simulink model "Thrustcontrol"  (R2015a)
settings: Solver=ode3  StartTime=0.0  StopTime=200  FixedStep=0.01  MaxStep=10.0  RelTol=1e-3
values from neighbouring files (symbols this model uses):
  C = [C1;C2;C3;C4;C5;C6]    [initfile.m]    (also in thrustallocationQuadraticFixed.m)
  D = 3.0/100    (= 0.03)    [initfile.m]    (also in thrustallocationQuadraticFixed.m = 0.0411111111111)
  eps_c = 3    [initfile.m]
  epsilon = 0.5    [initfile.m]    (also in thrustallocationPseudo.m = u(10); thrustallocationQuadraticFixed.m = u(10))
  hd = c2d(H1,0.01,'foh')    [initfile.m]
  hd2 = c2d(H2,0.01,'zoh')    [initfile.m]
  I_s = 25000 /747225    (= 0.0334571246947)    [initfile.m]
  k_cc = 1    [initfile.m]
  K_omega = 0.3    [initfile.m]
  Kp = 3.3    [initfile.m]
  Kq = 0.266    [initfile.m]
  Kqr = 0.266    [initfile.m]
  Kt = 0.445    [initfile.m]
  Ktr = 0.445    [initfile.m]
  Max_Acceleration = 5    [initfile.m]
  Max_rotation = 5*sqrt(lambda)    [initfile.m]
  Max_thrust = 0.12    [initfile.m]
  n_c = 5    [initfile.m]
  n_max = (lambda/sqrt(lambda))*170/1.4    [initfile.m]
  p_cc = 0.5    [initfile.m]
  P_max = 2*pi*n_max*Q_max    (= 239.439495498)    [initfile.m]
  pwm_to_shaft_coeff = coeffvalues(PWMToShaft)    [initfile.m]
  pwm_to_thrust_coeff = coeffvalues(PWMToForce)    [initfile.m]
  Q_f0 = 0.3    [initfile.m]
  Q_max = (Kq0*Rho_m*D^5*n_max^2*k)    (= 0.224164584)    [initfile.m]
  r = 0    [initfile.m]    (also in thrustallocationQuadraticFixed.m)
  r_cc = 2    [initfile.m]
  Rho = Rho_m    (= 1000)    [initfile.m]
  shaft_to_pwm_coeff = coeffvalues(ShaftToPWM)    [initfile.m]
  tc = [1;2;0.5]    [initfile.m]    (also in testgd.m = [-1,0,0]'; thrustallocationPseudo.m = [u(1),u(2),u(3)]'; thrustallocationQuadraticFixed.m = [u(1),u(2),u(3)]')
  Thrust_algorithm = 1    [initfile.m]
  thrust_to_pwm_coeff = coeffvalues(ForceToPWM)    [initfile.m]
  Thruster_control = 1    [initfile.m]
  Thruster_lock = 1    [initfile.m]
undefined symbols (not defined in the file or in its folder): Thruster
libraries: simulink x6, simulink_extras x3
(part 1 of 2)
settings Model: CovModelRefEnable=off  Creator=Preben  LastModifiedBy=Preben
settings SolverCC: AlgebraicLoopSolver=LineSearch
settings DataIOCC: SaveFormat=Dataset
settings HardwareCC: ProdBitPerPointer=64  ProdLargestAtomicFloat=Float  ProdIntDivRoundTo=Zero  ProdEndianess=LittleEndian  ProdHWDeviceType=Specified

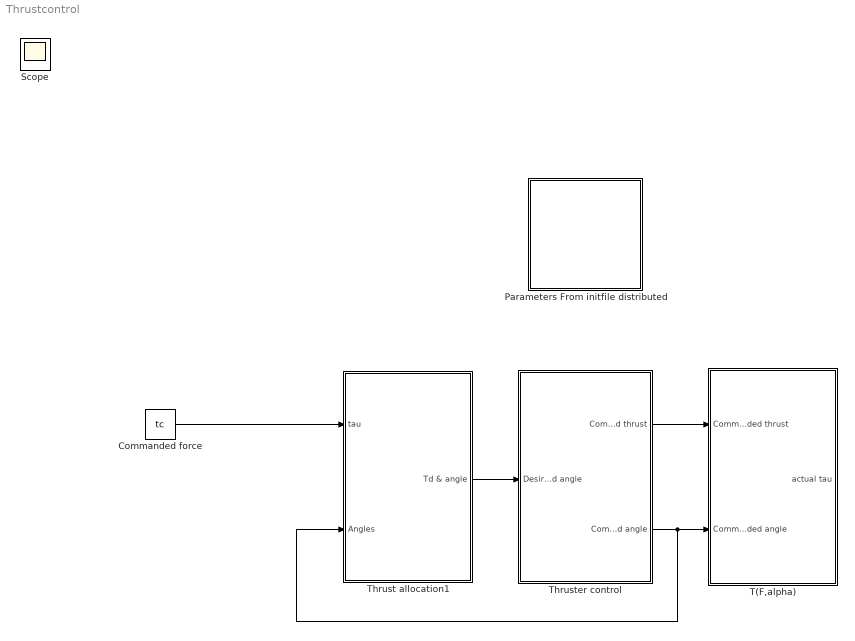
== system Thrustcontrol ==
  Commanded force : Constant  Value=tc
  "Parameters From initfile distributed " : Subsystem
  T(F,alpha) : Subsystem
  Thrust allocation1 : Subsystem
  "Thruster control " : Subsystem
  Scope : Scope
      settings: YMin=-10  YMax=10  SaveName=ScopeData2
  wires:
  "Thruster control "/2(Commanded angle) -> T(F,alpha)/2(Commanded angle), Thrust allocation1/2(Angles)
  Thrust allocation1/1(Td & angle) -> "Thruster control "/1("Desired thrust and angle ")
  "Thruster control "/1("Commanded thrust ") -> T(F,alpha)/1(Commanded thrust)
  Commanded force/1 -> Thrust allocation1/1(tau)

== system Thrustcontrol/Parameters From initfile distributed  ==
  note: Propulsion Control
  Constant : Constant  Value=eps_c
  Constant1 : Constant  Value=k_cc
  Constant2 : Constant  Value=p_cc
  Constant3 : Constant  Value=r_cc
  Constant4 : Constant  Value=eps
  Constant5 : Constant  Value=n_c
  D : Constant  Value=D
  Kq : Constant  Value=Kq
  Kqr : Constant  Value=Kqr
  Kt : Constant  Value=Kt
  Ktr : Constant  Value=Ktr
  Rho : Constant  Value=Rho
  tag scope: D=global, Kq=global, Kqr=global, Kt=global, Ktr=global, Rho=global, eps=global, eps_c=global, k_cc=global, n_c=global, p_cc=global, r_cc=global
  wires:
  Kq/1 -> [Kq]
  Kt/1 -> [Kt]
  D/1 -> [D]
  Rho/1 -> [Rho]
  Constant/1 -> [eps_c]
  Constant1/1 -> [k_cc]
  Constant2/1 -> [p_cc]
  Constant3/1 -> [r_cc]
  Constant4/1 -> [eps]
  Kqr/1 -> [Kqr]
  Ktr/1 -> [Ktr]
  Constant5/1 -> [n_c]

== system Thrustcontrol/T(F,alpha) ==
  Commanded thrust : Inport
  Commanded angle : Inport  Port=2
  Gain : Gain  Commented=through  Gain=-1
  MATLAB Function : MATLAB Function  TreatAsAtomicUnit=on
  Radians to Degrees : simulink_extras/Transformations/Radians to Degrees
  X-position Thruster : Constant  Value=[Thruster.T1(1) Thruster.T2(1) Thruster.T3(1) Thruster.T4(1) Thruster.T5(1) Thruster.T6(1)]
  Y-position Thruster : Constant  Value=[Thruster.T1(2) Thruster.T2(2) Thruster.T3(2) Thruster.T4(2) Thruster.T5(2) Thruster.T6(2)]
  actual tau : Outport
  wires:
  Commanded thrust/1 -> Gain/1
  Commanded angle/1 -> Radians to Degrees/1
  X-position Thruster/1 -> MATLAB Function/3(PosX)
  Y-position Thruster/1 -> MATLAB Function/4(PosY)
  MATLAB Function/1(actual_tau) -> actual tau/1
  Gain/1 -> MATLAB Function/1(thrust_actual)
  Radians to Degrees/1 -> MATLAB Function/2(alpha_actual)

== system Thrustcontrol/Thrust allocation1 ==
  tau : Inport
  Angles : Inport  Port=2
  "  Thrust calculated" : Selector  InputPortWidth=12  Indices=[7 8 9 10 11 12]
  " Angle calculated" : Selector  InputPortWidth=12  Indices=[1 2 3 4 5 6]
  Choosing Fixed / Azimuth angle : Switch  Threshold=1
  Choosing Fixed / Azimuth angle1 : Switch  Threshold=1
  Constant to avoid singularities : Constant  Value=eps
  For Each Subsystem : Subsystem  TreatAsAtomicUnit=on
  Mux : Mux  Inputs=3
  Mux1 : Mux  Inputs=2
  Mux2 : Mux  Inputs=2
  Radians to Degrees : simulink_extras/Transformations/Radians to Degrees
  Switch Azimuth/Fixed angles : Constant  Value=Thruster_lock
  Switch Thrust Algorithm : Constant  Value=Thrust_algorithm
  Thrust and angle specified : Selector  InputPortWidth=12  Indices=[7 1 8 2 9 3 10 4 11 5 12 6]
  ThrustAllocation_Pseudoinverse : S-Function  Commented=on  FunctionName=thrustallocationPseudo  Parameters=Thruster
      settings: AttributesFormatString=%<Commented>
  ThrustAllocation_Quadratic : S-Function  RequirementInfo="{}  %GIDa_450166d5_5ee3_4ab6_8a02_aaacf35750e7"  FunctionName=thrustallocationQuadraticFixed  Parameters=Thruster,C,r
      settings: AttributesFormatString=%<Commented>
  constant angle : Constant  Value=[Thruster.T1(3) Thruster.T2(3) Thruster.T3(3) Thruster.T4(3) Thruster.T5(3) Thruster.T6(3)]
  Td & angle : Outport
  wires:
  Switch Azimuth/Fixed angles/1 -> Choosing Fixed / Azimuth angle/2
  Constant to avoid singularities/1 -> Mux/3
  " Angle calculated"/1 -> Choosing Fixed / Azimuth angle/1
  Thrust and angle specified/1 -> Td & angle/1
  Mux2/1 -> Thrust and angle specified/1
  "  Thrust calculated"/1 -> Mux1/2, Mux2/2
  tau/1 -> Mux/1
  Choosing Fixed / Azimuth angle/1 -> For Each Subsystem/1(Desired Angle)
  Angles/1 -> Radians to Degrees/1
  For Each Subsystem/1("Out2 ") -> Mux2/1
  constant angle/1 -> For Each Subsystem/2("initial angle "), Choosing Fixed / Azimuth angle/3
  Radians to Degrees/1 -> Mux/2
  ThrustAllocation_Quadratic/1 -> Choosing Fixed / Azimuth angle1/1
  Switch Thrust Algorithm/1 -> Choosing Fixed / Azimuth angle1/2
  Choosing Fixed / Azimuth angle1/1 -> "  Thrust calculated"/1, " Angle calculated"/1
  ThrustAllocation_Pseudoinverse/1 -> Choosing Fixed / Azimuth angle1/3
  Mux1/1 -> ThrustAllocation_Quadratic/1
  Mux/1 -> Mux1/1, ThrustAllocation_Pseudoinverse/1

== system Thrustcontrol/Thruster control  ==
  "Desired thrust and angle " : Inport
  Demux : Demux  Outputs=12
  Mux : Mux  Inputs=12
  Mux1 : Mux  Inputs=2
  Selecting Desired thrust1 : Selector  InputPortWidth=12  Indices=[1 3 5 7 9 11]
  Selecting Desired thrust2 : Selector  InputPortWidth=12  Indices=[1 3 5 7 9 11]
  Selecting actual angle : Selector  InputPortWidth=12  Indices=[2 4 6 8 10 12]
  Subsystem : Subsystem
  Subsystem1 : Subsystem
  Thruster 1 : Subsystem
      settings: AttributesFormatString=%<MinAlgLoopOccurrences>
  Thruster 2 : Subsystem
      settings: AttributesFormatString=%<MinAlgLoopOccurrences>
  Thruster 3 : Subsystem
      settings: AttributesFormatString=%<MinAlgLoopOccurrences>
  Thruster 4 : Subsystem
      settings: AttributesFormatString=%<MinAlgLoopOccurrences>
  Thruster 5 : Subsystem
      settings: AttributesFormatString=%<MinAlgLoopOccurrences>
  Thruster 6 : Subsystem
      settings: AttributesFormatString=%<MinAlgLoopOccurrences>
  "Commanded thrust " : Outport
  Commanded angle : Outport  Port=2
  wires:
  Selecting actual angle/1 -> Subsystem1/1(Calculated angles)
  "Desired thrust and angle "/1 -> Selecting actual angle/1, Selecting Desired thrust1/1
  Subsystem1/1(Commanded angles) -> Commanded angle/1
  Subsystem/1(Thrust from model) -> "Commanded thrust "/1
  Mux/1 -> Selecting Desired thrust2/1
  Demux/1 -> Thruster 1/1(Desired thrust 1)
  Demux/2 -> Thruster 2/1(Desired thrust 1)
  Demux/3 -> Thruster 3/1(Desired thrust 1)
  Demux/4 -> Thruster 4/1(Desired thrust 1)
  Demux/5 -> Thruster 5/1(Desired thrust 1)
  Demux/6 -> Thruster 6/1(Desired thrust 1)
  Selecting Desired thrust1/1 -> Mux1/1
  Thruster 1/1("Commanded thrust ") -> Mux/1
  Thruster 1/2(Shaft speed) -> Mux/2
  Thruster 2/1("Commanded thrust ") -> Mux/3
  Thruster 3/1("Commanded thrust ") -> Mux/5
  Thruster 4/1("Commanded thrust ") -> Mux/7
  Thruster 5/1("Commanded thrust ") -> Mux/9
  Thruster 6/1("Commanded thrust ") -> Mux/11
  Thruster 2/2(Shaft speed) -> Mux/4
  Thruster 3/2(Shaft speed) -> Mux/6
  Thruster 4/2(Shaft speed) -> Mux/8
  Thruster 5/2(Shaft speed) -> Mux/10
  Thruster 6/2(Shaft speed) -> Mux/12
  Selecting Desired thrust2/1 -> Subsystem/1(Calculated thrust)
  Mux1/1 -> Demux/1
  Subsystem/2(pwm to shaftspeed) -> Mux1/2
  Demux/7 -> Thruster 1/2(shaft speed)
  Demux/8 -> Thruster 2/2(shaft speed)
  Demux/9 -> Thruster 3/2(shaft speed)
  Demux/10 -> Thruster 4/2(shaft speed)
  Demux/11 -> Thruster 5/2(shaft speed)
  Demux/12 -> Thruster 6/2(shaft speed)

== system Thrustcontrol/Thrust allocation1/For Each Subsystem ==
  Desired Angle : Inport  Partition=on  PartitionDimension=1  PartitionWidth=1
  "initial angle " : Inport  Port=2  Partition=on  PartitionDimension=1  PartitionWidth=1
  Degrees to Radians : simulink_extras/Transformations/Degrees to Radians
  Discrete-Time Integrator : DiscreteIntegrator  ExternalReset=either  InitialConditionSource=external  InitialConditionSetting=State (most efficient)  SampleTime=0.01  UpperSaturationLimit=180  LowerSaturationLimit=-180
  For Each : ForEach  DisableCoverage=on  IndexMode=One-based
  MATLAB Function : MATLAB Function  TreatAsAtomicUnit=on
  MATLAB Function1 : MATLAB Function  TreatAsAtomicUnit=on
  Max Rotation Rate : Saturate  UpperLimit=Max_rotation  LowerLimit=-Max_rotation
  constant : Constant  Value=0
  "Out2 " : Outport  ConcatenationDimension=1
  wires:
  Degrees to Radians/1 -> MATLAB Function/1(angle)
  MATLAB Function/1(y) -> "Out2 "/1
  Discrete-Time Integrator/1 -> Degrees to Radians/1, MATLAB Function1/2(actual)  "angle"
  "initial angle "/1 -> Discrete-Time Integrator/3
  Max Rotation Rate/1 -> Discrete-Time Integrator/1
  MATLAB Function1/1(psi_D) -> Max Rotation Rate/1
  Desired Angle/1 -> MATLAB Function1/1(desired)
  constant/1 -> Discrete-Time Integrator/2

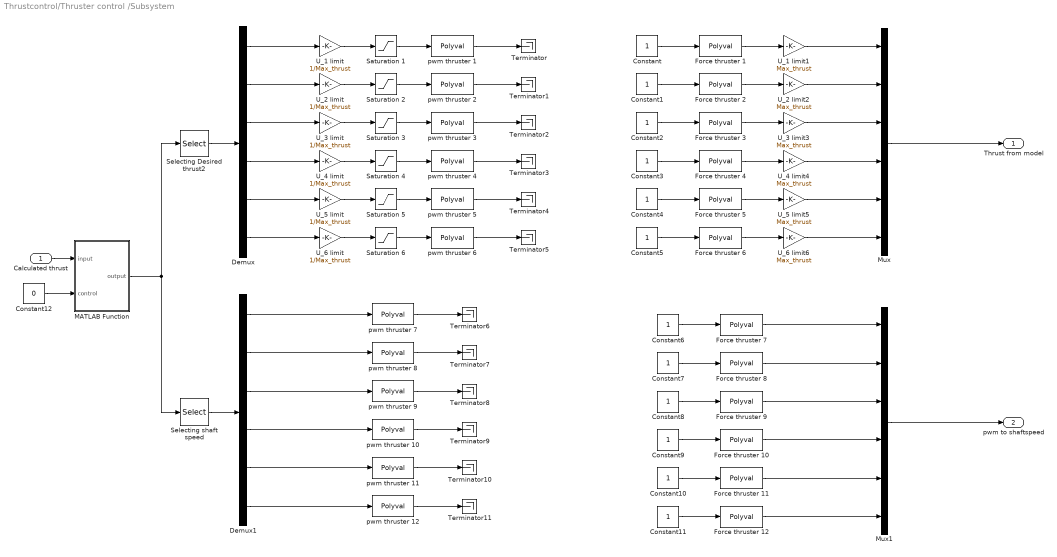
== system Thrustcontrol/Thruster control /Subsystem ==
  Calculated thrust : Inport
  Constant{,1..11} (12 alike) : Constant
  Constant12 : Constant  Value=0
  Demux : Demux  Outputs=6
  Demux1 : Demux  Outputs=6
  Force thruster {1..2,4..6} (5 alike) : Polyval  Coefs=pwm_to_thrust_coeff
  Force thruster {7..12} (6 alike) : Polyval  Coefs=pwm_to_shaft_coeff
  Force thruster 3 : Polyval  Coefs=thrust_to_pwm_coeff
  MATLAB Function : MATLAB Function  TreatAsAtomicUnit=on
  Mux : Mux  Inputs=6
  Mux1 : Mux  Inputs=6
  Saturation {1..6} (6 alike) : Saturate  UpperLimit=1  LowerLimit=-1
  Selecting Desired thrust2 : Selector  InputPortWidth=12  Indices=[1 3 5 7 9 11]
  Selecting shaft speed : Selector  InputPortWidth=12  Indices=[2 4 6 8 10 12]
  Terminator{,1..11} (12 alike) : Terminator
  U_1 limit : Gain  Gain=1/Max_thrust
  U_1 limit1 : Gain  Gain=Max_thrust
  U_2 limit : Gain  Gain=1/Max_thrust
  U_2 limit2 : Gain  Gain=Max_thrust
  U_3 limit : Gain  Gain=1/Max_thrust
  U_3 limit3 : Gain  Gain=Max_thrust
  U_4 limit : Gain  Gain=1/Max_thrust
  U_4 limit4 : Gain  Gain=Max_thrust
  U_5 limit : Gain  Gain=1/Max_thrust
  U_5 limit5 : Gain  Gain=Max_thrust
  U_6 limit : Gain  Gain=1/Max_thrust
  U_6 limit6 : Gain  Gain=Max_thrust
  pwm thruster {1..6} (6 alike) : Polyval  Coefs=thrust_to_pwm_coeff
  pwm thruster {7..12} (6 alike) : Polyval  Coefs=shaft_to_pwm_coeff
  Thrust from model : Outport
  pwm to shaftspeed : Outport  Port=2
  wires:
  Demux/1 -> U_1 limit/1
  U_1 limit/1 -> Saturation 1/1
  Demux/2 -> U_2 limit/1
  U_2 limit/1 -> Saturation 2/1
  Demux/3 -> U_3 limit/1
  U_3 limit/1 -> Saturation 3/1
  Demux/4 -> U_4 limit/1
  U_4 limit/1 -> Saturation 4/1
  Demux/5 -> U_5 limit/1
  U_5 limit/1 -> Saturation 5/1
  Demux/6 -> U_6 limit/1
  U_6 limit/1 -> Saturation 6/1
  Mux/1 -> Thrust from model/1
  U_1 limit1/1 -> Mux/1
  U_6 limit6/1 -> Mux/6
  U_5 limit5/1 -> Mux/5
  U_4 limit4/1 -> Mux/4
  U_3 limit3/1 -> Mux/3
  U_2 limit2/1 -> Mux/2
  Saturation 1/1 -> pwm thruster 1/1
  Saturation 6/1 -> pwm thruster 6/1
  Saturation 5/1 -> pwm thruster 5/1
  Saturation 4/1 -> pwm thruster 4/1
  Saturation 3/1 -> pwm thruster 3/1
  Saturation 2/1 -> pwm thruster 2/1
  pwm thruster 1/1 -> Terminator/1
  pwm thruster 6/1 -> Terminator5/1
  pwm thruster 5/1 -> Terminator4/1
  pwm thruster 4/1 -> Terminator3/1
  pwm thruster 3/1 -> Terminator2/1
  pwm thruster 2/1 -> Terminator1/1
  Force thruster 1/1 -> U_1 limit1/1
  Force thruster 6/1 -> U_6 limit6/1
  Force thruster 5/1 -> U_5 limit5/1
  Force thruster 2/1 -> U_2 limit2/1
  Force thruster 3/1 -> U_3 limit3/1
  Force thruster 4/1 -> U_4 limit4/1
  Constant/1 -> Force thruster 1/1
  Constant4/1 -> Force thruster 5/1
  Constant3/1 -> Force thruster 4/1
  Constant2/1 -> Force thruster 3/1
  Constant1/1 -> Force thruster 2/1
  Constant5/1 -> Force thruster 6/1
  MATLAB Function/1(output) -> Selecting Desired thrust2/1, Selecting shaft speed/1
  pwm thruster 7/1 -> Terminator6/1
  pwm thruster 12/1 -> Terminator11/1
  pwm thruster 11/1 -> Terminator10/1
  pwm thruster 10/1 -> Terminator9/1
  pwm thruster 9/1 -> Terminator8/1
  pwm thruster 8/1 -> Terminator7/1
  Demux1/1 -> pwm thruster 7/1
  Demux1/2 -> pwm thruster 8/1
  Demux1/3 -> pwm thruster 9/1
  Demux1/4 -> pwm thruster 10/1
  Demux1/5 -> pwm thruster 11/1
  Demux1/6 -> pwm thruster 12/1
  Mux1/1 -> pwm to shaftspeed/1
  Force thruster 7/1 -> Mux1/1
  Force thruster 12/1 -> Mux1/6
  Force thruster 11/1 -> Mux1/5
  Force thruster 10/1 -> Mux1/4
  Force thruster 9/1 -> Mux1/3
  Force thruster 8/1 -> Mux1/2
  Constant6/1 -> Force thruster 7/1
  Constant10/1 -> Force thruster 11/1
  Constant9/1 -> Force thruster 10/1
  Constant8/1 -> Force thruster 9/1
  Constant7/1 -> Force thruster 8/1
  Constant11/1 -> Force thruster 12/1
  Selecting Desired thrust2/1 -> Demux/1
  Selecting shaft speed/1 -> Demux1/1
  Calculated thrust/1 -> MATLAB Function/1(input)
  Constant12/1 -> MATLAB Function/2(control)

== system Thrustcontrol/Thruster control /Subsystem1 ==
  Calculated angles : Inport
  Demux : Demux  Outputs=6
  Mux : Mux  Inputs=6
  Saturation {1..6} (6 alike) : Saturate  UpperLimit=pi  LowerLimit=-pi
  Commanded angles : Outport
  wires:
  Calculated angles/1 -> Demux/1
  Demux/1 -> Saturation 1/1
  Demux/2 -> Saturation 2/1
  Demux/3 -> Saturation 3/1
  Demux/4 -> Saturation 4/1
  Demux/5 -> Saturation 5/1
  Demux/6 -> Saturation 6/1
  Mux/1 -> Commanded angles/1
  Saturation 1/1 -> Mux/1
  Saturation 6/1 -> Mux/6
  Saturation 5/1 -> Mux/5
  Saturation 2/1 -> Mux/2
  Saturation 3/1 -> Mux/3
  Saturation 4/1 -> Mux/4

== system Thrustcontrol/Thruster control /Thruster 1 ==
  Desired thrust 1 : Inport
  shaft speed : Inport  Port=2
  Constant : Constant  Value=hd2.den{1,1}
  Constant1 : Constant  Value=hd2.num{1,1}
  Discrete Transfer Fcn : DiscreteTransferFcn  NumeratorSource=Input port  DenominatorSource=Input port  Denominator=[0.2 1]  a0EqualsOne=on
      settings: InputPortMap=u0,p1,p3
  Losses (placeholder) : Constant  Value=0
  Propeller Hydrodynamics : Subsystem
  Shaft dynamics : Subsystem
  Thruster control : Subsystem
  "Commanded thrust " : Outport
  Shaft speed : Outport  Port=2
  wires:
  Losses (placeholder)/1 -> Propeller Hydrodynamics/1(env)
  Shaft dynamics/1(n) -> Shaft speed/1, Propeller Hydrodynamics/2(n)
  Propeller Hydrodynamics/2(Qa) -> Shaft dynamics/2(Qa)
  Desired thrust 1/1 -> Thruster control/1("T_d ")
  Propeller Hydrodynamics/1(Ta) -> "Commanded thrust "/1
  Thruster control/1(Qc) -> Discrete Transfer Fcn/1
  Constant1/1 -> Discrete Transfer Fcn/2
  Constant/1 -> Discrete Transfer Fcn/3
  Discrete Transfer Fcn/1 -> Shaft dynamics/1(Qm)
  shaft speed/1 -> Thruster control/2(n)

== system Thrustcontrol/Thruster control /Thruster 2 ==
  Desired thrust 1 : Inport
  shaft speed : Inport  Port=2
  Constant : Constant  Value=hd2.den{1,1}
  Constant1 : Constant  Value=hd2.num{1,1}
  Discrete Transfer Fcn : DiscreteTransferFcn  NumeratorSource=Input port  DenominatorSource=Input port  Denominator=[0.2 1]  SampleTime=0.01  a0EqualsOne=on
      settings: InputPortMap=u0,p1,p3
  Losses (placeholder) : Constant  Value=0
  Propeller Hydrodynamics : Subsystem
  Shaft dynamics : Subsystem
  Thruster control : Subsystem
  "Commanded thrust " : Outport
  Shaft speed : Outport  Port=2
  wires:
  Losses (placeholder)/1 -> Propeller Hydrodynamics/1(env)
  Shaft dynamics/1(n) -> Propeller Hydrodynamics/2(n), Shaft speed/1
  Propeller Hydrodynamics/2(Qa) -> Shaft dynamics/2(Qa)
  Thruster control/1(Qc) -> Discrete Transfer Fcn/1
  Discrete Transfer Fcn/1 -> Shaft dynamics/1(Qm)
  Desired thrust 1/1 -> Thruster control/1("T_d ")
  Propeller Hydrodynamics/1(Ta) -> "Commanded thrust "/1
  Constant1/1 -> Discrete Transfer Fcn/2
  Constant/1 -> Discrete Transfer Fcn/3
  shaft speed/1 -> Thruster control/2(n)

== system Thrustcontrol/Thruster control /Thruster 3 ==
  Desired thrust 1 : Inport
  shaft speed : Inport  Port=2
  Constant : Constant  Value=hd2.den{1,1}
  Constant1 : Constant  Value=hd2.num{1,1}
  Discrete Transfer Fcn : DiscreteTransferFcn  NumeratorSource=Input port  DenominatorSource=Input port  Denominator=[0.2 1]  SampleTime=0.01  a0EqualsOne=on
      settings: InputPortMap=u0,p1,p3
  Losses (placeholder) : Constant  Value=0
  Propeller Hydrodynamics : Subsystem
  Shaft dynamics : Subsystem
  Thruster control : Subsystem
  "Commanded thrust " : Outport
  Shaft speed : Outport  Port=2
  wires:
  Losses (placeholder)/1 -> Propeller Hydrodynamics/1(env)
  Shaft dynamics/1(n) -> Propeller Hydrodynamics/2(n), Shaft speed/1
  Propeller Hydrodynamics/2(Qa) -> Shaft dynamics/2(Qa)
  Thruster control/1(Qc) -> Discrete Transfer Fcn/1
  Discrete Transfer Fcn/1 -> Shaft dynamics/1(Qm)
  Desired thrust 1/1 -> Thruster control/1("T_d ")
  Propeller Hydrodynamics/1(Ta) -> "Commanded thrust "/1
  Constant1/1 -> Discrete Transfer Fcn/2
  Constant/1 -> Discrete Transfer Fcn/3
  shaft speed/1 -> Thruster control/2(n)

== system Thrustcontrol/Thruster control /Thruster 4 ==
  Desired thrust 1 : Inport
  shaft speed : Inport  Port=2
  Constant : Constant  Value=hd2.den{1,1}
  Constant1 : Constant  Value=hd2.num{1,1}
  Discrete Transfer Fcn : DiscreteTransferFcn  NumeratorSource=Input port  DenominatorSource=Input port  Denominator=[0.2 1]  SampleTime=0.01  a0EqualsOne=on
      settings: InputPortMap=u0,p1,p3
  Losses (placeholder) : Constant  Value=0
  Propeller Hydrodynamics : Subsystem
  Shaft dynamics : Subsystem
  Thruster control : Subsystem
  "Commanded thrust " : Outport
  Shaft speed : Outport  Port=2
  wires:
  Losses (placeholder)/1 -> Propeller Hydrodynamics/1(env)
  Shaft dynamics/1(n) -> Propeller Hydrodynamics/2(n), Shaft speed/1
  Propeller Hydrodynamics/2(Qa) -> Shaft dynamics/2(Qa)
  Thruster control/1(Qc) -> Discrete Transfer Fcn/1
  Discrete Transfer Fcn/1 -> Shaft dynamics/1(Qm)
  Desired thrust 1/1 -> Thruster control/1("T_d ")
  Propeller Hydrodynamics/1(Ta) -> "Commanded thrust "/1
  Constant1/1 -> Discrete Transfer Fcn/2
  Constant/1 -> Discrete Transfer Fcn/3
  shaft speed/1 -> Thruster control/2(n)

== system Thrustcontrol/Thruster control /Thruster 5 ==
  Desired thrust 1 : Inport
  shaft speed : Inport  Port=2
  Constant : Constant  Value=hd2.den{1,1}
  Constant1 : Constant  Value=hd2.num{1,1}
  Discrete Transfer Fcn : DiscreteTransferFcn  NumeratorSource=Input port  DenominatorSource=Input port  Denominator=[0.2 1]  SampleTime=0.01  a0EqualsOne=on
      settings: InputPortMap=u0,p1,p3
  Losses (placeholder) : Constant  Value=0
  Propeller Hydrodynamics : Subsystem
  Shaft dynamics : Subsystem
  Thruster control : Subsystem
  "Commanded thrust " : Outport
  Shaft speed : Outport  Port=2
  wires:
  Losses (placeholder)/1 -> Propeller Hydrodynamics/1(env)
  Shaft dynamics/1(n) -> Propeller Hydrodynamics/2(n), Shaft speed/1
  Propeller Hydrodynamics/2(Qa) -> Shaft dynamics/2(Qa)
  Thruster control/1(Qc) -> Discrete Transfer Fcn/1
  Discrete Transfer Fcn/1 -> Shaft dynamics/1(Qm)
  Desired thrust 1/1 -> Thruster control/1("T_d ")
  Propeller Hydrodynamics/1(Ta) -> "Commanded thrust "/1
  Constant1/1 -> Discrete Transfer Fcn/2
  Constant/1 -> Discrete Transfer Fcn/3
  shaft speed/1 -> Thruster control/2(n)

== system Thrustcontrol/Thruster control /Thruster 6 ==
  Desired thrust 1 : Inport
  shaft speed : Inport  Port=2
  Constant : Constant  Value=hd2.den{1,1}
  Constant1 : Constant  Value=hd2.num{1,1}
  Discrete Transfer Fcn : DiscreteTransferFcn  NumeratorSource=Input port  DenominatorSource=Input port  Denominator=[0.2 1]  SampleTime=0.01  a0EqualsOne=on
      settings: InputPortMap=u0,p1,p3
  Losses (placeholder) : Constant  Value=0
  Propeller Hydrodynamics : Subsystem
  Shaft dynamics : Subsystem
  Thruster control : Subsystem
  "Commanded thrust " : Outport
  Shaft speed : Outport  Port=2
  wires:
  Losses (placeholder)/1 -> Propeller Hydrodynamics/1(env)
  Shaft dynamics/1(n) -> Propeller Hydrodynamics/2(n), Shaft speed/1
  Propeller Hydrodynamics/2(Qa) -> Shaft dynamics/2(Qa)
  Thruster control/1(Qc) -> Discrete Transfer Fcn/1
  Discrete Transfer Fcn/1 -> Shaft dynamics/1(Qm)
  Desired thrust 1/1 -> Thruster control/1("T_d ")
  Propeller Hydrodynamics/1(Ta) -> "Commanded thrust "/1
  Constant1/1 -> Discrete Transfer Fcn/2
  Constant/1 -> Discrete Transfer Fcn/3
  shaft speed/1 -> Thruster control/2(n)

== system Thrustcontrol/Thruster control /Thruster 1/Propeller Hydrodynamics ==
  env : Inport
  n : Inport  Port=2
  Actual Force and Torque : MATLAB Function  TreatAsAtomicUnit=on
  Ta : Outport
  Qa : Outport  Port=2
  wires:
  n/1 -> Actual Force and Torque/1(n)
  [D] -> Actual Force and Torque/7(D)
  [Kq] -> Actual Force and Torque/2(Kq)
  Actual Force and Torque/2(Qa) -> Qa/1
  [Rho] -> Actual Force and Torque/6(Rho)
  env/1 -> Actual Force and Torque/9(env)
  [Kt] -> Actual Force and Torque/3(Kt)
  Actual Force and Torque/1(Ta) -> Ta/1
  [Ktr] -> Actual Force and Torque/4(Ktr)
  [Kqr] -> Actual Force and Torque/5(Kqr)
  [eps_c] -> Actual Force and Torque/8(eps_c)

== system Thrustcontrol/Thruster control /Thruster 1/Shaft dynamics ==
  Qm : Inport
  Qa : Inport  Port=2
  Constant : Constant  Value=0
  Discrete-Time Integrator : DiscreteIntegrator  ExternalReset=either  InitialConditionSetting=State (most efficient)  SampleTime=-1
  Finding rotation speed : Gain  Gain=1/(2*pi*I_s)
  K_omega : Gain  Gain=K_omega*2*pi
  Sum : Sum  Inputs=-+-
  n : Outport
  wires:
  Qm/1 -> Sum/2
  Sum/1 -> Finding rotation speed/1
  Qa/1 -> Sum/1
  K_omega/1 -> Sum/3
  Finding rotation speed/1 -> Discrete-Time Integrator/1
  Discrete-Time Integrator/1 -> n/1, K_omega/1
  Constant/1 -> Discrete-Time Integrator/2

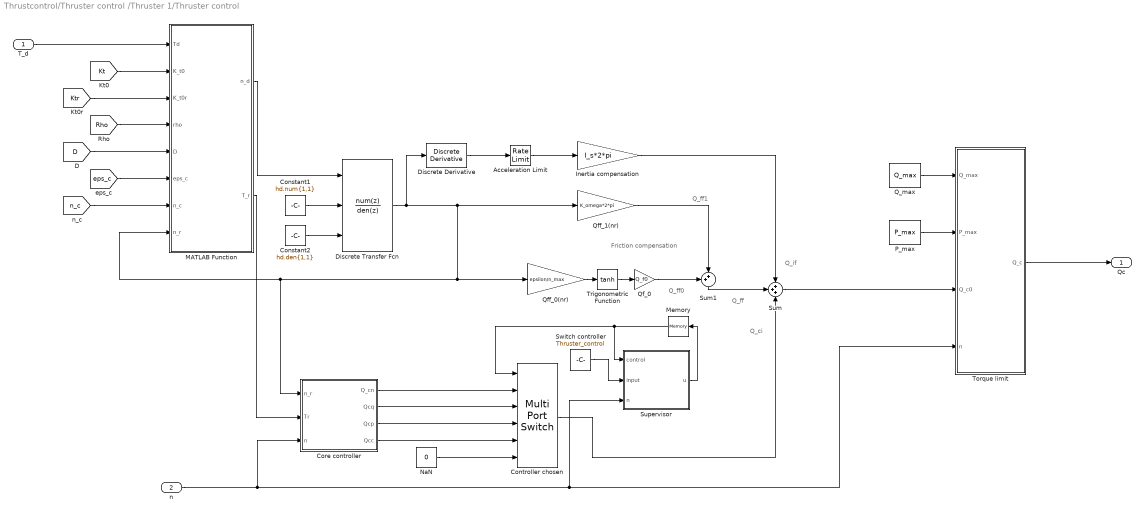
== system Thrustcontrol/Thruster control /Thruster 1/Thruster control ==
  note: Q_ci
  note: Q_if
  note: Q_ff
  note: Q_ff0
  note: Q_ff1
  note: Friction compensation
  "T_d " : Inport
  n : Inport  Port=2
  Acceleration Limit : RateLimiter  RisingSlewLimit=Max_Acceleration  FallingSlewLimit=-Max_Acceleration  SampleTimeMode=inherited
  Constant1 : Constant  Value=hd.num{1,1}  VectorParams1D=off
  Constant2 : Constant  Value=hd.den{1,1}  VectorParams1D=off
  Controller chosen : MultiPortSwitch  Inputs=5
  Core controller : Subsystem
  Discrete Transfer Fcn : DiscreteTransferFcn  NumeratorSource=Input port  Numerator=[8.76e-05 0.0003481 8.648e-05]  DenominatorSource=Input port  Denominator=[1 -1.974 0.9746]  SampleTime=0.01  a0EqualsOne=on
      settings: InputPortMap=u0,p1,p3
  Discrete Derivative : simulink/Discrete/Discrete Derivative  gainval=1.0  ICPrevScaledInput=0.0  InputProcessing=Inherited  OutMin=[]  OutMax=[]  OutDataType=fixdt(1, 16)  OutScaling=2^-10  DoSatur=off
  Inertia compensation : Gain  Gain=I_s*2*pi
  MATLAB Function : MATLAB Function  TreatAsAtomicUnit=on
  Memory : Memory  X0=1  InheritSampleTime=on
  NaN : Constant  Value=0
  P_max : Constant  Value=P_max
  Q_max : Constant  Value=Q_max
  Qf_0 : Gain  Gain=Q_f0
  Qff_0(nr) : Gain  Gain=epsilon/n_max
  Qff_1(nr) : Gain  Gain=K_omega*2*pi
  Sum : Sum  Inputs=+++
  Sum1 : Sum  Inputs=++|
  Supervisor : MATLAB Function  TreatAsAtomicUnit=on
  Switch controller : Constant  Value=Thruster_control
  Torque limit : MATLAB Function  TreatAsAtomicUnit=on
  Trigonometric Function : Trigonometry  Operator=tanh
  Qc : Outport
  wires:
  P_max/1 -> Torque limit/2(P_max)
  Q_max/1 -> Torque limit/1(Q_max)
  "T_d "/1 -> MATLAB Function/1(Td)
  [Kt] -> MATLAB Function/2(K_t0)
  [Rho] -> MATLAB Function/4(rho)
  [D] -> MATLAB Function/5(D)
  [eps_c] -> MATLAB Function/6(eps_c)
  MATLAB Function/2(T_r) -> Core controller/2("Tr ")
  MATLAB Function/1(n_d) -> Discrete Transfer Fcn/1
  Qff_0(nr)/1 -> Trigonometric Function/1
  Trigonometric Function/1 -> Qf_0/1
  NaN/1 -> Controller chosen/6
  Supervisor/1(u) -> Memory/1
  Memory/1 -> Controller chosen/1, Supervisor/1(control)
  Qff_1(nr)/1 -> Sum1/2
  Qf_0/1 -> Sum1/1
  Sum/1 -> Torque limit/3(Q_c0)
  Switch controller/1 -> Supervisor/2(input)
  Controller chosen/1 -> Sum/3
  Torque limit/1(Q_c) -> Qc/1
  Core controller/2(Qcq) -> Controller chosen/3
  Core controller/3(Qcp) -> Controller chosen/4
  Core controller/4(Qcc) -> Controller chosen/5
  Core controller/1(Q_cn) -> Controller chosen/2
  [Ktr] -> MATLAB Function/3(K_t0r)
  [n_c] -> MATLAB Function/7(n_c)
  Discrete Derivative/1 -> Acceleration Limit/1
  Sum1/1 -> Sum/2
  Constant1/1 -> Discrete Transfer Fcn/2
  Constant2/1 -> Discrete Transfer Fcn/3
  Inertia compensation/1 -> Sum/1
  n/1 -> Core controller/3("n "), Torque limit/4(n), Supervisor/3(n)
  Discrete Transfer Fcn/1 -> Core controller/1(n_r), MATLAB Function/8(n_r), Qff_0(nr)/1, Qff_1(nr)/1, Discrete Derivative/1
  Acceleration Limit/1 -> Inertia compensation/1

== system Thrustcontrol/Thruster control /Thruster 2/Propeller Hydrodynamics ==
  env : Inport
  n : Inport  Port=2
  Actual Force and Torque : MATLAB Function  TreatAsAtomicUnit=on
  Ta : Outport
  Qa : Outport  Port=2
  wires:
  n/1 -> Actual Force and Torque/1(n)
  [D] -> Actual Force and Torque/7(D)
  [Kq] -> Actual Force and Torque/2(Kq)
  Actual Force and Torque/2(Qa) -> Qa/1
  [Rho] -> Actual Force and Torque/6(Rho)
  env/1 -> Actual Force and Torque/9(env)
  [Kt] -> Actual Force and Torque/3(Kt)
  Actual Force and Torque/1(Ta) -> Ta/1
  [Ktr] -> Actual Force and Torque/4(Ktr)
  [Kqr] -> Actual Force and Torque/5(Kqr)
  [eps_c] -> Actual Force and Torque/8(eps_c)

== system Thrustcontrol/Thruster control /Thruster 2/Shaft dynamics ==
  Qm : Inport
  Qa : Inport  Port=2
  Constant : Constant  Value=0
  Discrete-Time Integrator : DiscreteIntegrator  ExternalReset=either  InitialConditionSetting=State (most efficient)  SampleTime=-1
  Finding rotation speed : Gain  Gain=1/(2*pi*I_s)
  K_omega : Gain  Gain=K_omega*2*pi
  Sum : Sum  Inputs=-+-
  n : Outport
  wires:
  Qm/1 -> Sum/2
  Sum/1 -> Finding rotation speed/1
  Qa/1 -> Sum/1
  K_omega/1 -> Sum/3
  Finding rotation speed/1 -> Discrete-Time Integrator/1
  Discrete-Time Integrator/1 -> K_omega/1, n/1
  Constant/1 -> Discrete-Time Integrator/2

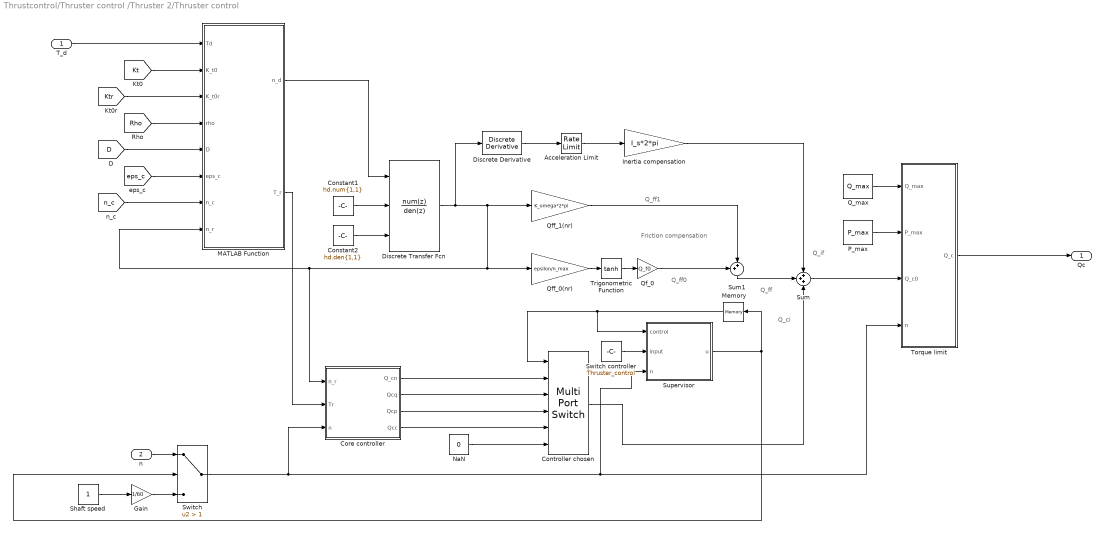
== system Thrustcontrol/Thruster control /Thruster 2/Thruster control ==
  note: Q_ci
  note: Q_if
  note: Q_ff
  note: Q_ff0
  note: Q_ff1
  note: Friction compensation
  "T_d " : Inport
  n : Inport  Port=2
  Acceleration Limit : RateLimiter  RisingSlewLimit=Max_Acceleration  FallingSlewLimit=-Max_Acceleration  SampleTimeMode=inherited
  Constant1 : Constant  Value=hd.num{1,1}  VectorParams1D=off
  Constant2 : Constant  Value=hd.den{1,1}  VectorParams1D=off
  Controller chosen : MultiPortSwitch  Inputs=5
  Core controller : Subsystem
  Discrete Transfer Fcn : DiscreteTransferFcn  NumeratorSource=Input port  Numerator=[8.76e-05 0.0003481 8.648e-05]  DenominatorSource=Input port  Denominator=[1 -1.974 0.9746]  SampleTime=0.01  a0EqualsOne=on
      settings: InputPortMap=u0,p1,p3
  Discrete Derivative : simulink/Discrete/Discrete Derivative  gainval=1.0  ICPrevScaledInput=0.0  InputProcessing=Inherited  OutMin=[]  OutMax=[]  OutDataType=fixdt(1, 16)  OutScaling=2^-10  DoSatur=off
  Gain : Gain  Gain=1/60
  Inertia compensation : Gain  Gain=I_s*2*pi
  MATLAB Function : MATLAB Function  TreatAsAtomicUnit=on
  Memory : Memory  X0=1
  NaN : Constant  Value=0
  P_max : Constant  Value=P_max
  Q_max : Constant  Value=Q_max
  Qf_0 : Gain  Gain=Q_f0
  Qff_0(nr) : Gain  Gain=epsilon/n_max
  Qff_1(nr) : Gain  Gain=K_omega*2*pi
  Shaft speed : Constant
  Sum : Sum  Inputs=+++
  Sum1 : Sum  Inputs=++|
  Supervisor : MATLAB Function  TreatAsAtomicUnit=on
  Switch : Switch  Criteria=u2 > Threshold  Threshold=1
  Switch controller : Constant  Value=Thruster_control
  Torque limit : MATLAB Function  TreatAsAtomicUnit=on
  Trigonometric Function : Trigonometry  Operator=tanh
  Qc : Outport
  wires:
  P_max/1 -> Torque limit/2(P_max)
  Q_max/1 -> Torque limit/1(Q_max)
  Torque limit/1(Q_c) -> Qc/1
  MATLAB Function/2(T_r) -> Core controller/2("Tr ")
  Qff_0(nr)/1 -> Trigonometric Function/1
  Trigonometric Function/1 -> Qf_0/1
  Sum1/1 -> Sum/2
  Core controller/1(Q_cn) -> Controller chosen/2
  Core controller/4(Qcc) -> Controller chosen/5
  NaN/1 -> Controller chosen/6
  Memory/1 -> Supervisor/1(control), Controller chosen/1
  Qff_1(nr)/1 -> Sum1/2
  Qf_0/1 -> Sum1/1
  Controller chosen/1 -> Sum/3
  Inertia compensation/1 -> Sum/1
  Sum/1 -> Torque limit/3(Q_c0)
  Core controller/3(Qcp) -> Controller chosen/4
  Core controller/2(Qcq) -> Controller chosen/3
  Switch controller/1 -> Supervisor/2(input)
  "T_d "/1 -> MATLAB Function/1(Td)
  [Kt] -> MATLAB Function/2(K_t0)
  [Rho] -> MATLAB Function/4(rho)
  [D] -> MATLAB Function/5(D)
  [eps_c] -> MATLAB Function/6(eps_c)
  [Ktr] -> MATLAB Function/3(K_t0r)
  [n_c] -> MATLAB Function/7(n_c)
  Constant1/1 -> Discrete Transfer Fcn/2
  Constant2/1 -> Discrete Transfer Fcn/3
  MATLAB Function/1(n_d) -> Discrete Transfer Fcn/1
  Discrete Derivative/1 -> Acceleration Limit/1
  Switch/1 -> Core controller/3("n "), Torque limit/4(n), Supervisor/3(n)
  Discrete Transfer Fcn/1 -> Discrete Derivative/1, Qff_0(nr)/1, Core controller/1(n_r), MATLAB Function/8(n_r), Qff_1(nr)/1
  Acceleration Limit/1 -> Inertia compensation/1
  Supervisor/1(u) -> Switch/2, Memory/1
  n/1 -> Switch/1
  Shaft speed/1 -> Gain/1
  Gain/1 -> Switch/3

== system Thrustcontrol/Thruster control /Thruster 3/Propeller Hydrodynamics ==
  env : Inport
  n : Inport  Port=2
  Actual Force and Torque : MATLAB Function  TreatAsAtomicUnit=on
  Ta : Outport
  Qa : Outport  Port=2
  wires:
  n/1 -> Actual Force and Torque/1(n)
  [D] -> Actual Force and Torque/7(D)
  [Kq] -> Actual Force and Torque/2(Kq)
  Actual Force and Torque/2(Qa) -> Qa/1
  [Rho] -> Actual Force and Torque/6(Rho)
  env/1 -> Actual Force and Torque/9(env)
  [Kt] -> Actual Force and Torque/3(Kt)
  Actual Force and Torque/1(Ta) -> Ta/1
  [Ktr] -> Actual Force and Torque/4(Ktr)
  [Kqr] -> Actual Force and Torque/5(Kqr)
  [eps_c] -> Actual Force and Torque/8(eps_c)

== system Thrustcontrol/Thruster control /Thruster 3/Shaft dynamics ==
  Qm : Inport
  Qa : Inport  Port=2
  Constant : Constant  Value=0
  Discrete-Time Integrator : DiscreteIntegrator  ExternalReset=either  InitialConditionSetting=State (most efficient)  SampleTime=-1
  Finding rotation speed : Gain  Gain=1/(2*pi*I_s)
  K_omega : Gain  Gain=K_omega*2*pi
  Sum : Sum  Inputs=-+-
  n : Outport
  wires:
  Qm/1 -> Sum/2
  Sum/1 -> Finding rotation speed/1
  Qa/1 -> Sum/1
  K_omega/1 -> Sum/3
  Finding rotation speed/1 -> Discrete-Time Integrator/1
  Discrete-Time Integrator/1 -> n/1, K_omega/1
  Constant/1 -> Discrete-Time Integrator/2

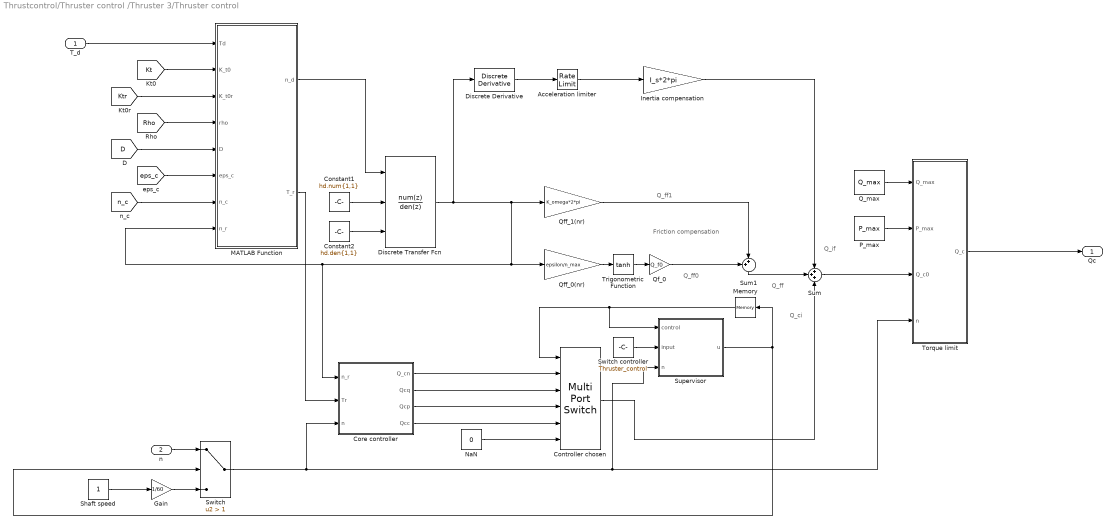
== system Thrustcontrol/Thruster control /Thruster 3/Thruster control ==
  note: Q_ci
  note: Q_if
  note: Q_ff
  note: Q_ff0
  note: Q_ff1
  note: Friction compensation
  "T_d " : Inport
  n : Inport  Port=2
  Acceleration limiter : RateLimiter  RisingSlewLimit=Max_Acceleration  FallingSlewLimit=-Max_Acceleration  SampleTimeMode=inherited
  Constant1 : Constant  Value=hd.num{1,1}  VectorParams1D=off
  Constant2 : Constant  Value=hd.den{1,1}  VectorParams1D=off
  Controller chosen : MultiPortSwitch  Inputs=5
  Core controller : Subsystem
  Discrete Transfer Fcn : DiscreteTransferFcn  NumeratorSource=Input port  Numerator=[8.76e-05 0.0003481 8.648e-05]  DenominatorSource=Input port  Denominator=[1 -1.974 0.9746]  SampleTime=0.01  a0EqualsOne=on
      settings: InputPortMap=u0,p1,p3
  Discrete Derivative : simulink/Discrete/Discrete Derivative  gainval=1.0  ICPrevScaledInput=0.0  InputProcessing=Inherited  OutMin=[]  OutMax=[]  OutDataType=fixdt(1, 16)  OutScaling=2^-10  DoSatur=off
  Gain : Gain  Gain=1/60
  Inertia compensation : Gain  Gain=I_s*2*pi
  MATLAB Function : MATLAB Function  TreatAsAtomicUnit=on
  Memory : Memory  X0=1
  NaN : Constant  Value=0
  P_max : Constant  Value=P_max
  Q_max : Constant  Value=Q_max
  Qf_0 : Gain  Gain=Q_f0
  Qff_0(nr) : Gain  Gain=epsilon/n_max
  Qff_1(nr) : Gain  Gain=K_omega*2*pi
  Shaft speed : Constant
  Sum : Sum  Inputs=+++
  Sum1 : Sum  Inputs=++|
  Supervisor : MATLAB Function  TreatAsAtomicUnit=on
  Switch : Switch  Criteria=u2 > Threshold  Threshold=1
  Switch controller : Constant  Value=Thruster_control
  Torque limit : MATLAB Function  TreatAsAtomicUnit=on
  Trigonometric Function : Trigonometry  Operator=tanh
  Qc : Outport
  wires:
  P_max/1 -> Torque limit/2(P_max)
  Q_max/1 -> Torque limit/1(Q_max)
  Torque limit/1(Q_c) -> Qc/1
  MATLAB Function/2(T_r) -> Core controller/2("Tr ")
  Discrete Derivative/1 -> Acceleration limiter/1
  Qff_0(nr)/1 -> Trigonometric Function/1
  Trigonometric Function/1 -> Qf_0/1
  Sum1/1 -> Sum/2
  Core controller/1(Q_cn) -> Controller chosen/2
  Core controller/4(Qcc) -> Controller chosen/5
  NaN/1 -> Controller chosen/6
  Memory/1 -> Supervisor/1(control), Controller chosen/1
  Qff_1(nr)/1 -> Sum1/2
  Qf_0/1 -> Sum1/1
  Controller chosen/1 -> Sum/3
  Inertia compensation/1 -> Sum/1
  Sum/1 -> Torque limit/3(Q_c0)
  Core controller/3(Qcp) -> Controller chosen/4
  Core controller/2(Qcq) -> Controller chosen/3
  Switch controller/1 -> Supervisor/2(input)
  "T_d "/1 -> MATLAB Function/1(Td)
  [Kt] -> MATLAB Function/2(K_t0)
  [Rho] -> MATLAB Function/4(rho)
  [D] -> MATLAB Function/5(D)
  [eps_c] -> MATLAB Function/6(eps_c)
  [Ktr] -> MATLAB Function/3(K_t0r)
  [n_c] -> MATLAB Function/7(n_c)
  Constant1/1 -> Discrete Transfer Fcn/2
  Constant2/1 -> Discrete Transfer Fcn/3
  MATLAB Function/1(n_d) -> Discrete Transfer Fcn/1
  Switch/1 -> Core controller/3("n "), Torque limit/4(n), Supervisor/3(n)
  Discrete Transfer Fcn/1 -> Discrete Derivative/1, Core controller/1(n_r), MATLAB Function/8(n_r), Qff_0(nr)/1, Qff_1(nr)/1
  Acceleration limiter/1 -> Inertia compensation/1
  Supervisor/1(u) -> Memory/1, Switch/2
  n/1 -> Switch/1
  Shaft speed/1 -> Gain/1
  Gain/1 -> Switch/3

== system Thrustcontrol/Thruster control /Thruster 4/Propeller Hydrodynamics ==
  env : Inport
  n : Inport  Port=2
  Actual Force and Torque : MATLAB Function  TreatAsAtomicUnit=on
  Ta : Outport
  Qa : Outport  Port=2
  wires:
  n/1 -> Actual Force and Torque/1(n)
  [D] -> Actual Force and Torque/7(D)
  [Kq] -> Actual Force and Torque/2(Kq)
  Actual Force and Torque/2(Qa) -> Qa/1
  [Rho] -> Actual Force and Torque/6(Rho)
  env/1 -> Actual Force and Torque/9(env)
  [Kt] -> Actual Force and Torque/3(Kt)
  Actual Force and Torque/1(Ta) -> Ta/1
  [Ktr] -> Actual Force and Torque/4(Ktr)
  [Kqr] -> Actual Force and Torque/5(Kqr)
  [eps_c] -> Actual Force and Torque/8(eps_c)

== system Thrustcontrol/Thruster control /Thruster 4/Shaft dynamics ==
  Qm : Inport
  Qa : Inport  Port=2
  Constant : Constant  Value=0
  Discrete-Time Integrator : DiscreteIntegrator  ExternalReset=either  InitialConditionSetting=State (most efficient)  SampleTime=-1
  Finding rotation speed : Gain  Gain=1/(2*pi*I_s)
  K_omega : Gain  Gain=K_omega*2*pi
  Sum : Sum  Inputs=-+-
  n : Outport
  wires:
  Qm/1 -> Sum/2
  Sum/1 -> Finding rotation speed/1
  Qa/1 -> Sum/1
  K_omega/1 -> Sum/3
  Finding rotation speed/1 -> Discrete-Time Integrator/1
  Discrete-Time Integrator/1 -> K_omega/1, n/1
  Constant/1 -> Discrete-Time Integrator/2

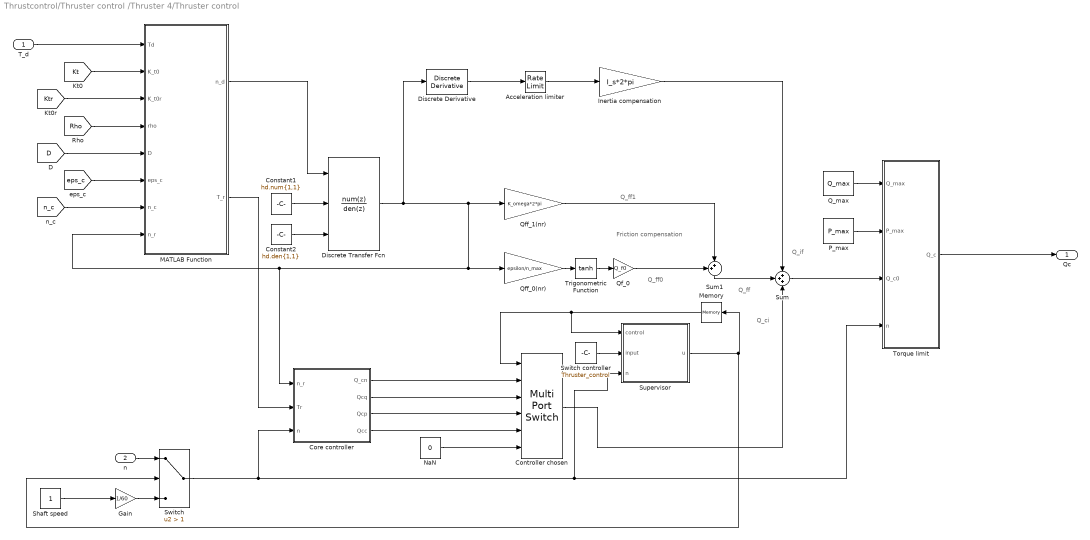
== system Thrustcontrol/Thruster control /Thruster 4/Thruster control ==
  note: Q_ci
  note: Q_if
  note: Q_ff
  note: Q_ff0
  note: Q_ff1
  note: Friction compensation
  "T_d " : Inport
  n : Inport  Port=2
  Acceleration limiter : RateLimiter  RisingSlewLimit=Max_Acceleration  FallingSlewLimit=-Max_Acceleration  SampleTimeMode=inherited
  Constant1 : Constant  Value=hd.num{1,1}  VectorParams1D=off
  Constant2 : Constant  Value=hd.den{1,1}  VectorParams1D=off
  Controller chosen : MultiPortSwitch  Inputs=5
  Core controller : Subsystem
  Discrete Transfer Fcn : DiscreteTransferFcn  NumeratorSource=Input port  Numerator=[8.76e-05 0.0003481 8.648e-05]  DenominatorSource=Input port  Denominator=[1 -1.974 0.9746]  SampleTime=0.01  a0EqualsOne=on
      settings: InputPortMap=u0,p1,p3
  Discrete Derivative : simulink/Discrete/Discrete Derivative  gainval=1.0  ICPrevScaledInput=0.0  InputProcessing=Inherited  OutMin=[]  OutMax=[]  OutDataType=fixdt(1, 16)  OutScaling=2^-10  DoSatur=off
  Gain : Gain  Gain=1/60
  Inertia compensation : Gain  Gain=I_s*2*pi
  MATLAB Function : MATLAB Function  TreatAsAtomicUnit=on
  Memory : Memory  X0=1
  NaN : Constant  Value=0
  P_max : Constant  Value=P_max
  Q_max : Constant  Value=Q_max
  Qf_0 : Gain  Gain=Q_f0
  Qff_0(nr) : Gain  Gain=epsilon/n_max
  Qff_1(nr) : Gain  Gain=K_omega*2*pi
  Shaft speed : Constant
  Sum : Sum  Inputs=+++
  Sum1 : Sum  Inputs=++|
  Supervisor : MATLAB Function  TreatAsAtomicUnit=on
  Switch : Switch  Criteria=u2 > Threshold  Threshold=1
  Switch controller : Constant  Value=Thruster_control
  Torque limit : MATLAB Function  TreatAsAtomicUnit=on
  Trigonometric Function : Trigonometry  Operator=tanh
  Qc : Outport
  wires:
  P_max/1 -> Torque limit/2(P_max)
  Q_max/1 -> Torque limit/1(Q_max)
  Torque limit/1(Q_c) -> Qc/1
  MATLAB Function/2(T_r) -> Core controller/2("Tr ")
  Discrete Derivative/1 -> Acceleration limiter/1
  Qff_0(nr)/1 -> Trigonometric Function/1
  Trigonometric Function/1 -> Qf_0/1
  Sum1/1 -> Sum/2
  Core controller/1(Q_cn) -> Controller chosen/2
  Core controller/4(Qcc) -> Controller chosen/5
  NaN/1 -> Controller chosen/6
  Memory/1 -> Supervisor/1(control), Controller chosen/1
  Qff_1(nr)/1 -> Sum1/2
  Qf_0/1 -> Sum1/1
  Controller chosen/1 -> Sum/3
  Inertia compensation/1 -> Sum/1
  Sum/1 -> Torque limit/3(Q_c0)
  Core controller/3(Qcp) -> Controller chosen/4
  Core controller/2(Qcq) -> Controller chosen/3
  Switch controller/1 -> Supervisor/2(input)
  "T_d "/1 -> MATLAB Function/1(Td)
  [Kt] -> MATLAB Function/2(K_t0)
  [Rho] -> MATLAB Function/4(rho)
  [D] -> MATLAB Function/5(D)
  [eps_c] -> MATLAB Function/6(eps_c)
  [Ktr] -> MATLAB Function/3(K_t0r)
  [n_c] -> MATLAB Function/7(n_c)
  Constant1/1 -> Discrete Transfer Fcn/2
  Constant2/1 -> Discrete Transfer Fcn/3
  MATLAB Function/1(n_d) -> Discrete Transfer Fcn/1
  Switch/1 -> Torque limit/4(n), Supervisor/3(n), Core controller/3("n ")
  Discrete Transfer Fcn/1 -> Discrete Derivative/1, Core controller/1(n_r), MATLAB Function/8(n_r), Qff_0(nr)/1, Qff_1(nr)/1
  Acceleration limiter/1 -> Inertia compensation/1
  Supervisor/1(u) -> Switch/2, Memory/1
  n/1 -> Switch/1
  Shaft speed/1 -> Gain/1
  Gain/1 -> Switch/3

== system Thrustcontrol/Thruster control /Thruster 5/Propeller Hydrodynamics ==
  env : Inport
  n : Inport  Port=2
  Actual Force and Torque : MATLAB Function  TreatAsAtomicUnit=on
  Ta : Outport
  Qa : Outport  Port=2
  wires:
  n/1 -> Actual Force and Torque/1(n)
  [D] -> Actual Force and Torque/7(D)
  [Kq] -> Actual Force and Torque/2(Kq)
  Actual Force and Torque/2(Qa) -> Qa/1
  [Rho] -> Actual Force and Torque/6(Rho)
  env/1 -> Actual Force and Torque/9(env)
  [Kt] -> Actual Force and Torque/3(Kt)
  Actual Force and Torque/1(Ta) -> Ta/1
  [Ktr] -> Actual Force and Torque/4(Ktr)
  [Kqr] -> Actual Force and Torque/5(Kqr)
  [eps_c] -> Actual Force and Torque/8(eps_c)

== system Thrustcontrol/Thruster control /Thruster 5/Shaft dynamics ==
  Qm : Inport
  Qa : Inport  Port=2
  Constant : Constant  Value=0
  Discrete-Time Integrator : DiscreteIntegrator  ExternalReset=either  InitialConditionSetting=State (most efficient)  SampleTime=-1
  Finding rotation speed : Gain  Gain=1/(2*pi*I_s)
  K_omega : Gain  Gain=K_omega*2*pi
  Sum : Sum  Inputs=-+-
  n : Outport
  wires:
  Qm/1 -> Sum/2
  Sum/1 -> Finding rotation speed/1
  Qa/1 -> Sum/1
  K_omega/1 -> Sum/3
  Finding rotation speed/1 -> Discrete-Time Integrator/1
  Discrete-Time Integrator/1 -> K_omega/1, n/1
  Constant/1 -> Discrete-Time Integrator/2

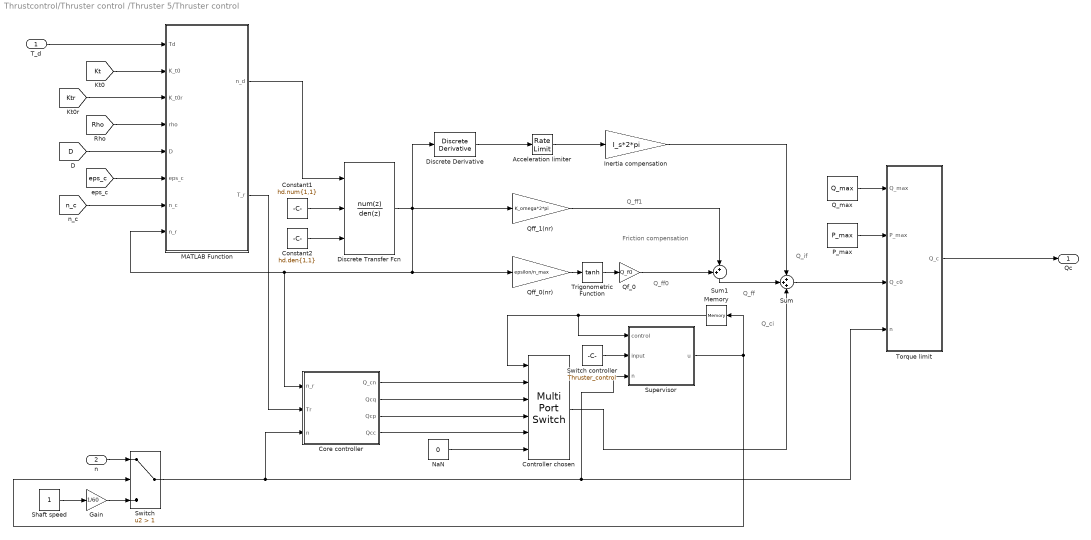
== system Thrustcontrol/Thruster control /Thruster 5/Thruster control ==
  note: Q_ci
  note: Q_if
  note: Q_ff
  note: Q_ff0
  note: Q_ff1
  note: Friction compensation
  "T_d " : Inport
  n : Inport  Port=2
  Acceleration limiter : RateLimiter  RisingSlewLimit=Max_Acceleration  FallingSlewLimit=-Max_Acceleration  SampleTimeMode=inherited
  Constant1 : Constant  Value=hd.num{1,1}  VectorParams1D=off
  Constant2 : Constant  Value=hd.den{1,1}  VectorParams1D=off
  Controller chosen : MultiPortSwitch  Inputs=5
  Core controller : Subsystem
  Discrete Transfer Fcn : DiscreteTransferFcn  NumeratorSource=Input port  Numerator=[8.76e-05 0.0003481 8.648e-05]  DenominatorSource=Input port  Denominator=[1 -1.974 0.9746]  SampleTime=0.01  a0EqualsOne=on
      settings: InputPortMap=u0,p1,p3
  Discrete Derivative : simulink/Discrete/Discrete Derivative  gainval=1.0  ICPrevScaledInput=0.0  InputProcessing=Inherited  OutMin=[]  OutMax=[]  OutDataType=fixdt(1, 16)  OutScaling=2^-10  DoSatur=off
  Gain : Gain  Gain=1/60
  Inertia compensation : Gain  Gain=I_s*2*pi
  MATLAB Function : MATLAB Function  TreatAsAtomicUnit=on
  Memory : Memory  X0=1
  NaN : Constant  Value=0
  P_max : Constant  Value=P_max
  Q_max : Constant  Value=Q_max
  Qf_0 : Gain  Gain=Q_f0
  Qff_0(nr) : Gain  Gain=epsilon/n_max
  Qff_1(nr) : Gain  Gain=K_omega*2*pi
  Shaft speed : Constant
  Sum : Sum  Inputs=+++
  Sum1 : Sum  Inputs=++|
  Supervisor : MATLAB Function  TreatAsAtomicUnit=on
  Switch : Switch  Criteria=u2 > Threshold  Threshold=1
  Switch controller : Constant  Value=Thruster_control
  Torque limit : MATLAB Function  TreatAsAtomicUnit=on
  Trigonometric Function : Trigonometry  Operator=tanh
  Qc : Outport
  wires:
  P_max/1 -> Torque limit/2(P_max)
  Q_max/1 -> Torque limit/1(Q_max)
  Torque limit/1(Q_c) -> Qc/1
  MATLAB Function/2(T_r) -> Core controller/2("Tr ")
  Discrete Derivative/1 -> Acceleration limiter/1
  Qff_0(nr)/1 -> Trigonometric Function/1
  Trigonometric Function/1 -> Qf_0/1
  Sum1/1 -> Sum/2
  Core controller/1(Q_cn) -> Controller chosen/2
  Core controller/4(Qcc) -> Controller chosen/5
  NaN/1 -> Controller chosen/6
  Memory/1 -> Supervisor/1(control), Controller chosen/1
  Qff_1(nr)/1 -> Sum1/2
  Qf_0/1 -> Sum1/1
  Controller chosen/1 -> Sum/3
  Inertia compensation/1 -> Sum/1
  Sum/1 -> Torque limit/3(Q_c0)
  Core controller/3(Qcp) -> Controller chosen/4
  Core controller/2(Qcq) -> Controller chosen/3
  Switch controller/1 -> Supervisor/2(input)
  "T_d "/1 -> MATLAB Function/1(Td)
  [Kt] -> MATLAB Function/2(K_t0)
  [Rho] -> MATLAB Function/4(rho)
  [D] -> MATLAB Function/5(D)
  [eps_c] -> MATLAB Function/6(eps_c)
  [Ktr] -> MATLAB Function/3(K_t0r)
  [n_c] -> MATLAB Function/7(n_c)
  Constant1/1 -> Discrete Transfer Fcn/2
  Constant2/1 -> Discrete Transfer Fcn/3
  MATLAB Function/1(n_d) -> Discrete Transfer Fcn/1
  Switch/1 -> Torque limit/4(n), Supervisor/3(n), Core controller/3("n ")
  Discrete Transfer Fcn/1 -> Discrete Derivative/1, Qff_0(nr)/1, Core controller/1(n_r), MATLAB Function/8(n_r), Qff_1(nr)/1
  Acceleration limiter/1 -> Inertia compensation/1
  Supervisor/1(u) -> Memory/1, Switch/2
  n/1 -> Switch/1
  Shaft speed/1 -> Gain/1
  Gain/1 -> Switch/3

== system Thrustcontrol/Thruster control /Thruster 6/Propeller Hydrodynamics ==
  env : Inport
  n : Inport  Port=2
  Actual Force and Torque : MATLAB Function  TreatAsAtomicUnit=on
  Ta : Outport
  Qa : Outport  Port=2
  wires:
  n/1 -> Actual Force and Torque/1(n)
  [D] -> Actual Force and Torque/7(D)
  [Kq] -> Actual Force and Torque/2(Kq)
  Actual Force and Torque/2(Qa) -> Qa/1
  [Rho] -> Actual Force and Torque/6(Rho)
  env/1 -> Actual Force and Torque/9(env)
  [Kt] -> Actual Force and Torque/3(Kt)
  Actual Force and Torque/1(Ta) -> Ta/1
  [Ktr] -> Actual Force and Torque/4(Ktr)
  [Kqr] -> Actual Force and Torque/5(Kqr)
  [eps_c] -> Actual Force and Torque/8(eps_c)

== system Thrustcontrol/Thruster control /Thruster 6/Shaft dynamics ==
  Qm : Inport
  Qa : Inport  Port=2
  Constant : Constant  Value=0
  Discrete-Time Integrator : DiscreteIntegrator  ExternalReset=either  InitialConditionSetting=State (most efficient)  SampleTime=-1
  Finding rotation speed : Gain  Gain=1/(2*pi*I_s)
  K_omega : Gain  Gain=K_omega*2*pi
  Sum : Sum  Inputs=-+-
  n : Outport
  wires:
  Qm/1 -> Sum/2
  Sum/1 -> Finding rotation speed/1
  Qa/1 -> Sum/1
  K_omega/1 -> Sum/3
  Finding rotation speed/1 -> Discrete-Time Integrator/1
  Discrete-Time Integrator/1 -> K_omega/1, n/1
  Constant/1 -> Discrete-Time Integrator/2

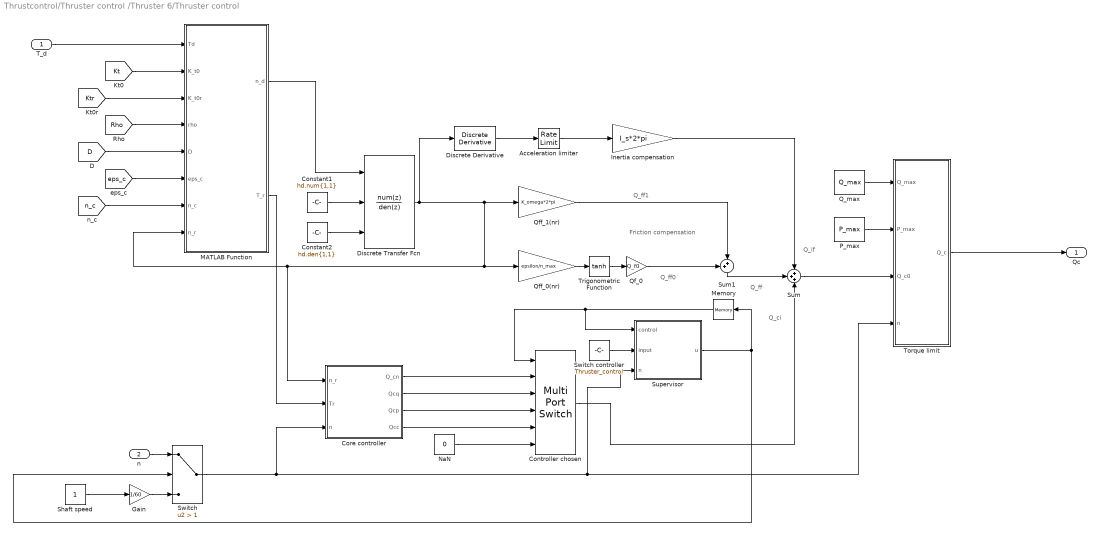
== system Thrustcontrol/Thruster control /Thruster 6/Thruster control ==
  note: Q_ci
  note: Q_if
  note: Q_ff
  note: Q_ff0
  note: Q_ff1
  note: Friction compensation
  "T_d " : Inport
  n : Inport  Port=2
  Acceleration limiter : RateLimiter  RisingSlewLimit=Max_Acceleration  FallingSlewLimit=-Max_Acceleration  SampleTimeMode=inherited
  Constant1 : Constant  Value=hd.num{1,1}  VectorParams1D=off
  Constant2 : Constant  Value=hd.den{1,1}  VectorParams1D=off
  Controller chosen : MultiPortSwitch  Inputs=5
  Core controller : Subsystem
  Discrete Transfer Fcn : DiscreteTransferFcn  NumeratorSource=Input port  Numerator=[8.76e-05 0.0003481 8.648e-05]  DenominatorSource=Input port  Denominator=[1 -1.974 0.9746]  SampleTime=0.01  a0EqualsOne=on
      settings: InputPortMap=u0,p1,p3
  Discrete Derivative : simulink/Discrete/Discrete Derivative  gainval=1.0  ICPrevScaledInput=0.0  InputProcessing=Inherited  OutMin=[]  OutMax=[]  OutDataType=fixdt(1, 16)  OutScaling=2^-10  DoSatur=off
  Gain : Gain  Gain=1/60
  Inertia compensation : Gain  Gain=I_s*2*pi
  MATLAB Function : MATLAB Function  TreatAsAtomicUnit=on
  Memory : Memory  X0=1
  NaN : Constant  Value=0
  P_max : Constant  Value=P_max
  Q_max : Constant  Value=Q_max
  Qf_0 : Gain  Gain=Q_f0
  Qff_0(nr) : Gain  Gain=epsilon/n_max
  Qff_1(nr) : Gain  Gain=K_omega*2*pi
  Shaft speed : Constant
  Sum : Sum  Inputs=+++
  Sum1 : Sum  Inputs=++|
  Supervisor : MATLAB Function  TreatAsAtomicUnit=on
  Switch : Switch  Criteria=u2 > Threshold  Threshold=1
  Switch controller : Constant  Value=Thruster_control
  Torque limit : MATLAB Function  TreatAsAtomicUnit=on
  Trigonometric Function : Trigonometry  Operator=tanh
  Qc : Outport
  wires:
  P_max/1 -> Torque limit/2(P_max)
  Q_max/1 -> Torque limit/1(Q_max)
  Torque limit/1(Q_c) -> Qc/1
  MATLAB Function/2(T_r) -> Core controller/2("Tr ")
  Discrete Derivative/1 -> Acceleration limiter/1
  Qff_0(nr)/1 -> Trigonometric Function/1
  Trigonometric Function/1 -> Qf_0/1
  Sum1/1 -> Sum/2
  Core controller/1(Q_cn) -> Controller chosen/2
  Core controller/4(Qcc) -> Controller chosen/5
  NaN/1 -> Controller chosen/6
  Memory/1 -> Supervisor/1(control), Controller chosen/1
  Qff_1(nr)/1 -> Sum1/2
  Qf_0/1 -> Sum1/1
  Controller chosen/1 -> Sum/3
  Inertia compensation/1 -> Sum/1
  Sum/1 -> Torque limit/3(Q_c0)
  Core controller/3(Qcp) -> Controller chosen/4
  Core controller/2(Qcq) -> Controller chosen/3
  Switch controller/1 -> Supervisor/2(input)
  "T_d "/1 -> MATLAB Function/1(Td)
  [Kt] -> MATLAB Function/2(K_t0)
  [Rho] -> MATLAB Function/4(rho)
  [D] -> MATLAB Function/5(D)
  [eps_c] -> MATLAB Function/6(eps_c)
  [Ktr] -> MATLAB Function/3(K_t0r)
  [n_c] -> MATLAB Function/7(n_c)
  Constant1/1 -> Discrete Transfer Fcn/2
  Constant2/1 -> Discrete Transfer Fcn/3
  MATLAB Function/1(n_d) -> Discrete Transfer Fcn/1
  Switch/1 -> Torque limit/4(n), Supervisor/3(n), Core controller/3("n ")
  Discrete Transfer Fcn/1 -> Discrete Derivative/1, Core controller/1(n_r), MATLAB Function/8(n_r), Qff_0(nr)/1, Qff_1(nr)/1
  Acceleration limiter/1 -> Inertia compensation/1
  Supervisor/1(u) -> Memory/1, Switch/2
  n/1 -> Switch/1
  Shaft speed/1 -> Gain/1
  Gain/1 -> Switch/3
